simulink model "Projekat_pod_a_simulink"  (R2024b)
settings: Solver=VariableStepAuto  StartTime=0.0  StopTime=1  RelTol=1e-3
settings Model: Creator=HP  LastModifiedBy=HP

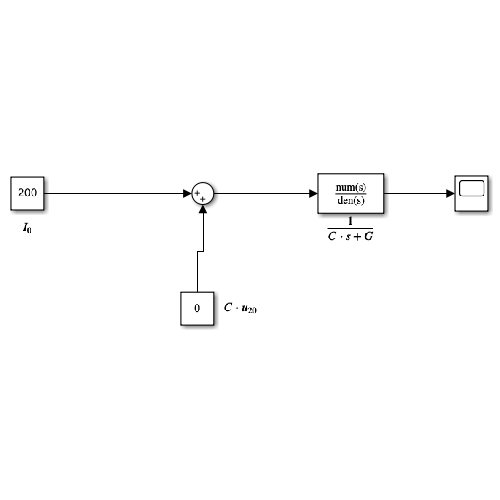
[thumbnail: Simulink's stored preview of the top-level diagram]
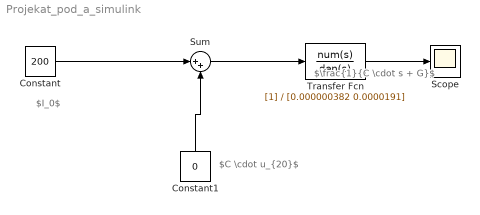
== system Projekat_pod_a_simulink ==
  note: $\frac{1}{C \cdot s + G}$
  note: $C \cdot u_{20}$
  note: $I_0$
  Constant : Constant  Value=200
  Constant1 : Constant  Value=0
  Scope : Scope
  Sum : Sum  Inputs=|++
  Transfer Fcn : TransferFcn  Denominator=[0.000000382 0.0000191]
  wires:
  Sum/1 -> Transfer Fcn/1
  Constant/1 -> Sum/1
  Constant1/1 -> Sum/2
  Transfer Fcn/1 -> Scope/1
